simulink model "ssc_auto_ev_20b"  (R2020b)
settings: Solver=VariableStepAuto  StartTime=0.0  StopTime=200  RelTol=1e-3  AbsTol=1e-3
PreLoadFcn:
  | % Simulation parameters
  | dt = 0.01;
  | 
  | % Battery cell parameters
  | ssc_lithium_cell_1RC_ini
  | Nseries = 100;
  | Nparallel = 10;
  | 
  | % Motor parameters
  | max_torque = 220;
  | max_power = 80e3;
  | 
  | % Vehicle parameters
  | vehicle_mass = 4000;
  | wheel_radius = 0.35;
  | area = 5;
  | drag_coefficient = 0.25;
  | air_density = 1.225;
  | gravity = 9.81;
  | rolling_res_ratio = 0.015;
  | 
  | % Differential drive parameters
  | gear_ratio = 12;
  | 
  | % Simplified braking system parameters
  | force_max_pedal = 500;
  | braking_torque_to_pedal_force_ratio = -16;
  | 
  | % Vehicle controller parameters
  | hill_hold_max_speed = 0.5;
  | 
  | % Water properties for cooling circuit
  | load WaterProperties
  | 
  | % Input signals for Signal Editor block
  | load ssc_auto_ev_Inputs
values from neighbouring files (symbols this model uses):
  C1_LUT = [1913.6 4625.7 23306 10736 18036 12251 9022.9 12447 18872 40764 18721 33630 ... (21 elements, 7x3)]    [ssc_auto_ev_param.mat]
  Capacity_LUT = [28.0081 27.625 27.6392]    [ssc_auto_ev_param.mat]
  cell_Cp_heat = 810.5328    [ssc_auto_ev_param.mat]
  cell_mass = 1    [ssc_auto_ev_param.mat]
  Em_LUT = [3.4966 3.5519 3.6183 3.7066 3.9131 4.0748 4.1923 3.5057 3.566 3.6337 3.7127 3.9259 ... (21 elements, 7x3)]    [ssc_auto_ev_param.mat]
  Qe_init = 15.6845    [ssc_auto_ev_param.mat]
  R0_LUT = [0.0117 0.011 0.0114 0.0107 0.0107 0.0113 0.0116 0.0085 0.0085 0.0087 0.0082 0.0083 ... (21 elements, 7x3)]    [ssc_auto_ev_param.mat]
  R1_LUT = [0.0109 0.0069 0.0047 0.0034 0.0033 0.0033 0.0028 0.0029 0.0024 0.0026 0.0016 0.0023 ... (21 elements, 7x3)]    [ssc_auto_ev_param.mat]
  SOC_LUT = [0 0.1 0.25 0.5 0.75 0.9 1]    [ssc_auto_ev_param.mat]
  T_init = 293.15    [ssc_auto_ev_param.mat]
  Temperature_LUT = [278.15 293.15 313.15]    [ssc_auto_ev_param.mat]
undefined symbols (not defined in the file or in its folder): DiscIntNeverNeededParam, K, Lambda, tau, x0
libraries: fl_lib x656, nesl_utility x86, simulink x21, LiBatteryElements_lib x16, SignalEditorBlockLib x4, simulink_extras x4
(part 1 of 13)
CloseFcn:
  | try,close(h1_ssc_auto_ev),end
  | clear h1_ssc_auto_ev
  | 
  | clear simlog_ssc_auto_ev
  | clear logsout_ssc_auto_ev
  | clear Nseries Nparallel
  | clear C1_LUT Capacity_LUT Cp Cv
  | clear Em_LUT Qe_init R0_LUT R1_LUT
  | clear SOC_LUT T T_init Temperature_LUT
  | clear air_density alpha area beta
  | clear braking_torque_to_pedal_force_ratio
  | clear cell_Cp_heat cell_area cell_height
  | clear cell_mass cell_rho_Cp cell_thickness
  | clear cell_volume cell_width drag_coefficient
  | clear dt force_max_pedal gear_ratio gravity
  | clear h h_conv hill_hold_max_speed k
  | clear max_power max_torque nu p rho
  | clear rolling_res_ratio simlog_TMotor tout u
  | clear vehicle_mass wheel_radius Test_1
Description:
  | Configuring an EV Simulation for Multirate HIL
settings Model: Creator=The MathWorks, Inc.  LastModifiedBy=amyyang
settings SolverCC: AutoScaleAbsTol=off
settings DataIOCC: ReturnWorkspaceOutputs=off  SignalLoggingName=logsout_ssc_auto_ev
settings DebuggingCC: SymbolicDimsDataTypeCodeGenerationDiagnostic=none
settings SFSimCC: CustomCodeUndefinedFunction=UseInterfaceOnly
settings SimscapeCC: SimscapeLogType=all  SimscapeLogName=simlog_ssc_auto_ev  SimscapeLogDataHistory=40000

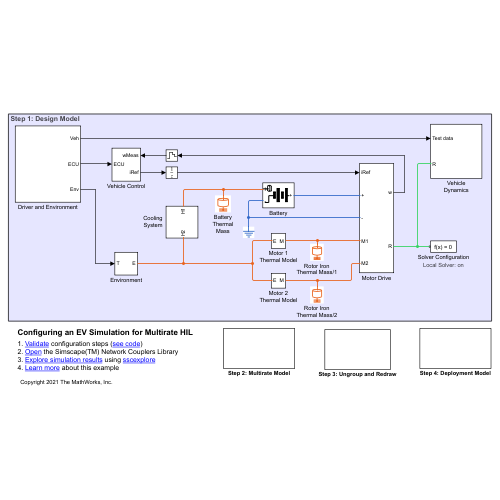
[thumbnail: Simulink's stored preview of the top-level diagram]
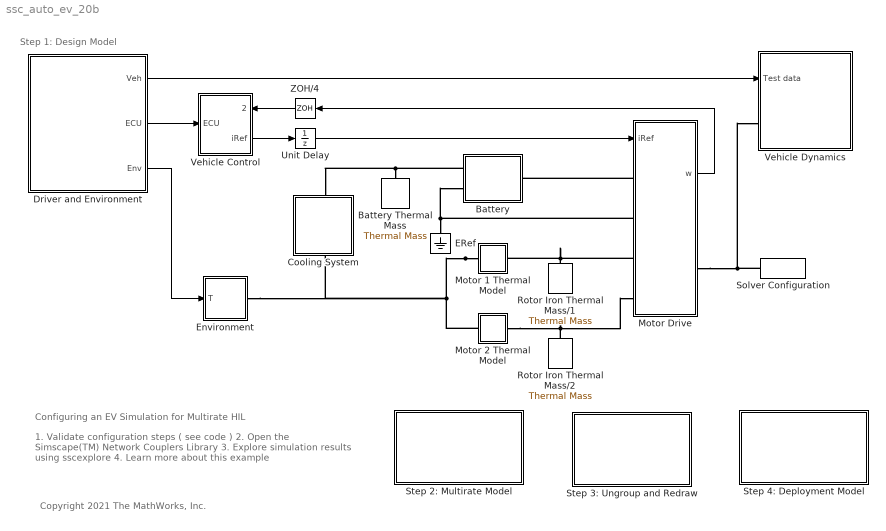
== system ssc_auto_ev_20b ==
  note: Step 1: Design Model
  note: Configuring an EV Simulation for Multirate HIL
  note: 1. Validate configuration steps ( see code )
      | 2. Open the Simscape(TM) Network Couplers Library
      | 3. Explore simulation results using sscexplore
      | 4. Learn more about this example
  note: Copyright 2021 The MathWorks, Inc.
  Battery : Subsystem  mask(Lithium cell (one RC-branch equivalent circuit)){Nseries=Nseries, Nparallel=Nparallel, Qe_init=Qe_init, Capacity_LUT=Capacity_LUT, Em_LUT=Em_LUT, R0_LUT=R0_LUT, R1_LUT=R1_LUT, C1_LUT=C1_LUT, SOC_LUT=SOC_LUT, Temperature_LUT=Temperature_LUT}
      mask prompts: Nseries "Number of series-connected parallel sets"; Nparallel "Number of parallel-connected cells per parallel set"; Qe_init "Initial cell charge deficit (A*hr)"; Capacity_LUT "Capacity (A*hr, 1xN table)"; Em_LUT "Em open-circuit voltage, Em (volts, MxN table)"; R0_LUT "R0 terminal resistance (ohms, MxN table)"; R1_LUT "R1 cell resistance (ohms, MxN table)"; C1_LUT "C1 capacitance (farads, MxN table)"; SOC_LUT "SOC table breakpoints (Mx1 array)"; Temperature_LUT "Temperature table breakpoints (K, 1xN array)"
      mask DialogControl ParameterTabVar0 Prompt: Main
      mask DialogControl ParameterTabVar01 Prompt: Electrical (per cell)
      mask DialogControl ParameterTabVar0123 Prompt: Table Breakpoints
      mask Display:
      | % Battery icon
      | plot([1.8 1.3],[0 0])
      | plot([-0.6 -1.6 -1.6 -2.2],[0 0 -0.9 -0.9])
      | patch([1 1 -1 -1]*0.15+0.7,[-1 1 1 -1]*0.4,[0;0;0]);
      | patch([1 1 -1 -1]*0.15-0.6,[-1 1 1 -1]*0.4,[0;0;0]);
      | patch([1 1 -1 -1]*0.15+1.3,[-1 1 1 -1]*0.8,[0;0;0]);
      | patch([1 1 -1 -1]*0.15-0.0,[-1 1 1 -1]*0.8,[0;0;0]);
      | % Thermal port
      | plot([-1.6,-1.3],[1.2,1.2])
      | plot([-1.6,-1.3],[0.5,0.5])
      | plot([-1.6,-2.5],[0.8,0.8])
      | plot(0.2*sin(0:2*pi/50:2*pi)-1.6,0.35*cos(0:2*pi/50:2*pi)+0.85)
      | plot(0.2*sin(0:2*pi/50:pi)-1.3,0.35*cos(0:2*pi/50:pi)+0.85)
      | 
      | % Plot points to set plot range
      | color('white');plot(2.5,1.5);plot(-2.5,-1.5)
  Battery Thermal Mass : fl_lib/Thermal/Thermal Elements/Thermal Mass  mass=cell_mass*Nseries*Nparallel kg  sp_heat=cell_Cp_heat J/(K*kg)  T_specify=on  T_priority=High  T=T_init K  T_nominal_specify=off  T_nominal_unit=K  T_nominal_value=1  Q_specify=off  Q_priority=None  Q=0 W  Q_nominal_specify=off  Q_nominal_unit=W  Q_nominal_value=1
      settings: SourceProductBaseCode=PW,SS,VE
  Cooling System : Subsystem  Tag=PublishSubsystem
      settings: PortSchema="{\"entries\":[{\"content\":{\"sides\":[{\"content\":{\"connectorIds\":[]},\"type\":\"ConnectorPlacement.EquallySpacedRectSide\",\"uuid\":\"d96bbf63-bcbb-4f3a-92bd-eaf78ab4538b\"},{\"content\":{\"connectorIds\":[],\"side\":\"RIGHT\"},\"type\":\"ConnectorPlacement.EquallySpacedRectSide\",\"uuid\":\"b082d3d3-6635-4bf9-9df2-69e4bab78a2b\"},{\"content\":{\"connectorIds\":[\"LConn1\"],\"side\":\"TOP\"},\"type\":\"ConnectorPlacement.EquallySpacedRectSide\",\"uuid\":\"f7177de9-9ba4-478b-b096-87cbc5cd4871\"},{\"content\":{\"connectorIds\":[\"RConn1\"],\"side\":\"BOTTOM\"},\"type\":\"ConnectorPlacement.EquallySpacedRectSide\",\"uuid\":\"4233a269-bfd6-4033-b1ed-0dae7bb50bca\"}]},\"type\":\"ConnectorPlacement.EquallySpacedConnector\",\"uuid\":\"6f10551f-62c9-4564-9ac9-7ef3b87c77d6\"}],\"packageUris\":[\"http://schema.mathworks.com/mf0/Connector/R2020b\"],\"version\":\"1.0\"}"
  Driver and Environment : Subsystem
  ERef : fl_lib/Electrical/Electrical Elements/Electrical Reference
      settings: SourceProductBaseCode=PW,SS,VE
  Environment : Subsystem
  Motor 1 Thermal Model : Subsystem
  Motor 2 Thermal Model : Subsystem
  Motor Drive : Subsystem  Tag=PublishSubsystem  VariantControl=Variant1
  Rotor Iron Thermal Mass/1 : fl_lib/Thermal/Thermal Elements/Thermal Mass  mass=10 kg  sp_heat=447 J/(K*kg)  T_specify=on  T_priority=High  T=T_init K  T_nominal_specify=off  T_nominal_unit=K  T_nominal_value=1  Q_specify=off  Q_priority=None  Q=0 W  Q_nominal_specify=off  Q_nominal_unit=W  Q_nominal_value=1
      settings: SourceProductBaseCode=PW,SS,VE
  Rotor Iron Thermal Mass/2 : fl_lib/Thermal/Thermal Elements/Thermal Mass  mass=10 kg  sp_heat=447 J/(K*kg)  T_specify=on  T_priority=High  T=T_init K  T_nominal_specify=off  T_nominal_unit=K  T_nominal_value=1  Q_specify=off  Q_priority=None  Q=0 W  Q_nominal_specify=off  Q_nominal_unit=W  Q_nominal_value=1
      settings: SourceProductBaseCode=PW,SS,VE
  Solver Configuration : nesl_utility/Solver Configuration  PhysicalDomain=network_engine_domain  SubClassName=solver  LeftPortType=input  RightPortType=generic  Tones=[]  Harmonics=[]  SimulateNoise=off  Profile=off  UseLocalSampling=off  EnableSwitchedLinearOptims=on  FrequencyDomain=off  UseCCode=off  RelTol=0.001  AbsTol=1e-06  MinStep=1e-09  ToWorkspace=off  RevertToSquareIcSolve=off  NumHomotopyIterations=100  PhasorMode=off  PhasorModeNumHarmonics=1  DoDC=off  ResidualTolerance=1e-9  UseLocalSolver=on  LocalSolverChoice=NE_BACKWARD_EULER_ADVANCER  LocalSolverSampleTime=dt  DoFixedCost=on  MaxNonlinIter=3  MaxModeIter=2  ComputeImpulses=off  ImpulseIterations=2  LinearAlgebra=auto  EquationFormulation=NE_TIME_EF  DelaysMemoryBudget=1024  AutomaticFiltering=on  FilteringTimeConstant=0.001  PartitionStorageMethod=AS_NEEDED  PartitionMemoryBudget=1024  PartitionMethod=FAST
      settings: AttributesFormatString=Local Solver: %<UseLocalSolver>  SourceProductBaseCode=SS,PW,VE
  Step 2: Multirate Model : Subsystem
  Step 3: Ungroup and Redraw : Subsystem
  Step 4: Deployment Model : Subsystem
  Unit Delay : UnitDelay  SampleTime=dt  HasFrameUpgradeWarning=on
  Vehicle Dynamics : Subsystem
  Vehicle Control : Subsystem  Tag=PublishSubsystem
      settings: PortSchema="{\"entries\":[{\"content\":{\"sides\":[{\"content\":{\"connectorIds\":[\"In1\"]},\"type\":\"ConnectorPlacement.EquallySpacedRectSide\",\"uuid\":\"b68a5c30-2a17-4a0c-a85e-064518f12190\"},{\"content\":{\"connectorIds\":[\"In2\",\"Out1\"],\"side\":\"RIGHT\"},\"type\":\"ConnectorPlacement.EquallySpacedRectSide\",\"uuid\":\"e14e894a-37e1-47c1-8ef8-e46ccf22e5bb\"},{\"content\":{\"connectorIds\":[],\"side\":\"TOP\"},\"type\":\"ConnectorPlacement.EquallySpacedRectSide\",\"uuid\":\"6e722464-54b7-4a5f-a776-dae3a11285e7\"}]},\"type\":\"ConnectorPlacement.EquallySpacedConnector\",\"uuid\":\"82601a10-23cc-4178-a2d7-02b0e1b6e975\"}],\"packageUris\":[\"http://schema.mathworks.com/mf0/Connector/R2020b\"],\"version\":\"1.0\"}"
  ZOH/4 : ZeroOrderHold  SampleTime=dt
  wires:
  Motor Drive/1(w) -> ZOH/4/1
  Unit Delay/1 -> Motor Drive/1(iRef)
  Vehicle Control/1(iRef) -> Unit Delay/1
  ZOH/4/1 -> Vehicle Control/2(wMeas)
  Driver and Environment/2(ECU) -> Vehicle Control/1(ECU)
  Driver and Environment/3(Env) -> Environment/1(T)
  Driver and Environment/1(Veh) -> Vehicle Dynamics/1(Test data)
  connections:
  Motor 1 Thermal Model/LConn1 -- Motor 2 Thermal Model/LConn1 -- Environment/RConn1 -- Cooling System/RConn1
  Motor Drive/LConn2 -- Battery/LConn2 -- ERef/LConn1
  Motor Drive/LConn1 -- Battery/RConn1
  Motor Drive/RConn1 -- Vehicle Dynamics/LConn1 -- Solver Configuration/RConn1
  Motor Drive/LConn3 -- Motor 1 Thermal Model/RConn1 -- Rotor Iron Thermal Mass/1/LConn1
  Battery/LConn1 -- Cooling System/LConn1 -- Battery Thermal Mass/LConn1
  Motor 2 Thermal Model/RConn1 -- Rotor Iron Thermal Mass/2/LConn1 -- Motor Drive/LConn4

== system ssc_auto_ev_20b/Battery ==
  note: Scale up voltage drop to total
      | of Ns series-connected cells
  Controlled Voltage Source : fl_lib/Electrical/Electrical Sources/Controlled Voltage Source
      settings: SourceProductBaseCode=PW,SS,VE
  Electric and Thermal Model : Subsystem  Tag=PublishSubsystem
  Nseries-1 : fl_lib/Physical Signals/Functions/PS Gain  gain=Nseries-1
      settings: SourceProductBaseCode=PW,SS,VE
  PS Terminator : fl_lib/Physical Signals/Sinks/PS Terminator
      settings: SourceProductBaseCode=PW,SS,VE
  Temperature Sensor : fl_lib/Thermal/Thermal Sensors/Temperature Sensor
      settings: SourceProductBaseCode=PW,SS,VE
  Thermal Reference : fl_lib/Thermal/Thermal Elements/Thermal Reference
      settings: SourceProductBaseCode=PW,SS,VE
  Voltage Sensor : fl_lib/Electrical/Electrical Sensors/Voltage Sensor
      settings: SourceProductBaseCode=PW,SS,VE
  + : PMIOPort  Tag=PMCPort  Side=Right
  H : PMIOPort  Tag=PMCPort  Port=2  Side=Left
  - : PMIOPort  Tag=PMCPort  Port=3  Side=Left
  connections:
  H/RConn1 -- Temperature Sensor/LConn1 -- Electric and Thermal Model/LConn1
  Controlled Voltage Source/LConn1 -- Voltage Sensor/RConn2 -- Electric and Thermal Model/RConn2
  Nseries-1/LConn1 -- Voltage Sensor/RConn1
  Voltage Sensor/LConn1 -- Electric and Thermal Model/RConn1 -- +/RConn1
  Nseries-1/RConn1 -- Controlled Voltage Source/RConn1
  Controlled Voltage Source/RConn2 -- -/RConn1
  Temperature Sensor/RConn1 -- Thermal Reference/LConn1
  PS Terminator/LConn1 -- Temperature Sensor/RConn2

== system ssc_auto_ev_20b/Cooling System ==
  note: Radiator
  note: Battery Heat Exchanger
  " Heat Exchanger Characteristic" : Subsystem
  Convection Battery-Env : fl_lib/Thermal/Thermal Elements/Convective Heat Transfer  area=cell_area m^2  heat_tr_coeff=h_conv W/(m^2 * K)  T_specify=off  T_priority=High  T=0 K  T_nominal_specify=off  T_nominal_unit=K  T_nominal_value=1  Q_specify=off  Q_priority=High  Q=0 J/s  Q_nominal_specify=off  Q_nominal_unit=J/s  Q_nominal_value=1
      settings: SourceProductBaseCode=PW,SS,VE
  Expansion Tank : Subsystem
  Heat Exchanger Characteristic : Subsystem
  Hose Radiator : fl_lib/Thermal Liquid/Elements/Pipe (TL)  length=2000 mm  area=pi*25^2 mm^2  Dh=50 mm  length_add=500 mm  roughness=1.5e-5 m  Re_lam=2e+3  Re_tur=4e+3  shape_factor=64  Nu_lam=3.66  dynamic_compressibility=1  inertia=0  p0=1 atm  T0=20 degC  mdot0=0.1 kg/s
      settings: SourceProductBaseCode=PW,SS,VE
  Hose Inlet : fl_lib/Thermal Liquid/Elements/Pipe (TL)  length=500 mm  area=pi*25^2 mm^2  Dh=50 mm  length_add=500 mm  roughness=1.5e-5 m  Re_lam=2e+3  Re_tur=4e+3  shape_factor=64  Nu_lam=3.66  dynamic_compressibility=1  inertia=0  p0=1 atm  T0=20 degC  mdot0=0.1 kg/s
      settings: SourceProductBaseCode=PW,SS,VE
  Hose Outlet : fl_lib/Thermal Liquid/Elements/Pipe (TL)  length=500 mm  area=pi*25^2 mm^2  Dh=50 mm  length_add=500 mm  roughness=1.5e-5 m  Re_lam=2e+3  Re_tur=4e+3  shape_factor=64  Nu_lam=3.66  dynamic_compressibility=1  inertia=0  p0=1 atm  T0=20 degC  mdot0=0.1 kg/s
      settings: SourceProductBaseCode=PW,SS,VE
  Insulator Inlet Hose : fl_lib/Thermal/Thermal Elements/Perfect Insulator  T_specify=off  T_priority=High  T=0 K  T_nominal_specify=off  T_nominal_unit=K  T_nominal_value=1
      settings: SourceProductBaseCode=PW,SS,VE
  Insulator Outlet Hose : fl_lib/Thermal/Thermal Elements/Perfect Insulator  T_specify=off  T_priority=High  T=0 K  T_nominal_specify=off  T_nominal_unit=K  T_nominal_value=1
      settings: SourceProductBaseCode=PW,SS,VE
  PS Terminator : fl_lib/Physical Signals/Sinks/PS Terminator
      settings: SourceProductBaseCode=PW,SS,VE
  Pipe : fl_lib/Thermal Liquid/Elements/Pipe (TL)  length=400 mm  area=pi*25^2 mm^2  Dh=50 mm  length_add=500 mm  roughness=1.5e-5 m  Re_lam=2e+3  Re_tur=4e+3  shape_factor=64  Nu_lam=3.66  dynamic_compressibility=1  inertia=0  p0=1 atm  T0=20 degC  mdot0=0.1 kg/s
      settings: SourceProductBaseCode=PW,SS,VE
  Pump : fl_lib/Thermal Liquid/Sources/Mass Flow Rate Source (TL)  commanded_mass_flow=0.2 kg/s  area=pi*25^2 mm^2
      settings: SourceProductBaseCode=PW,SS,VE  InternalSimscapePortConfiguration="{\"Bottom\":[],\"Left\":[{\"id\":\"A\",\"label\":\"A\",\"type\":\"foundation.thermal_liquid.thermal_liquid\"}],\"Right\":[{\"id\":\"B\",\"label\":\"B\",\"type\":\"foundation.thermal_liquid.thermal_liquid\"}],\"Top\":[]}"
  Sensing Inlet Temperature : Subsystem
      mask Display: disp('T');
  Sensing Temperature : Subsystem
      mask Display: disp('T')
  Thermal Liquid Settings (TL) : fl_lib/Thermal Liquid/Utilities/Thermal Liquid Settings (TL)  table_dimensions=0  T_TLU=T K  p_TLU=p Pa  p_atm=1 atm  pT_region_flag=0  T_min=273.16 K  T_max=373.16 K  p_min=0.1 bar  p_max=500 bar  T_min_1D=273.16 K  T_max_1D=373.16 K  p_min_1D=0.01 MPa  p_max_1D=50 MPa  pT_validity_TLU=ones(11, 12)  rho_parameterization_2D=1  rho_parameterization_1D=1  rho_TLU=rho kg/m^3  beta_TLU=beta Pa  alpha_TLU=alpha 1/K  rho_TLU_2=[999.7973, 999.8431, 1002.3216, 1004.8218, 1007.293, 1009.7358, 1012.1506, 1014.5379, 1016.8979, 1019.2311, 1021.538, 1023.8188; 999.6579, 999.7009, 1002.0303, 1004.382, 1006.7084, 1009.0101, 1011.2874, 1013.5407, 1015.7703, 1017.9766, 1020.1599, 1022.3206; 998.1632, 998.2045, 1000.4375, 1002.6924, 1004.9239, 1007.1324, 1009.3183, 1011.4819, 1013.6236, 1015.7438, 1017.8428, 1019.921; 995.6057, 995.6458, 997.81864, 1000.0128, 1002.1841, 1004.3332, 1006.4603, 1008.566, 1010.6505, 1012.7144, 1014.758, 1016.7815; 992.1724, 992.2119, 994.35133, 996.5113, 998.6484, 1000.7633, 1002.8563, 1004.928, 1006.9788, 1009.009, 1011.0192, 1013.0097; 988.02, 988.0299, 990.15684, 992.3035, 994.4268, 996.5273, 998.6056, 1000.6622, 1002.6976, 1004.7123, 1006.7067, 1008.6813; 983.18, 983.1901, 985.3217, 987.4721, 989.5983, 991.7008, 993.7803, 995.8374, 997.8726, 999.8864, 1001.8795, 1003.8522; 977.75, 977.7583, 979.9094, 982.0783, 984.2216, 986.34, 988.4343, 990.505, 992.5529, 994.5786, 996.5825, 998.5654; 971.77, 971.7836, 973.96734, 976.1678, 978.3409, 980.4876, 982.6087, 984.7049, 986.7768, 988.8254, 990.8511, 992.8545; 965.26, 965.3023, 967.53107, 969.7753, 971.9901, 974.1764, 976.3354, 978.4676, 980.5741, 982.6556, 984.7129, 986.7465; 958.62, 958.6315, 960.627, 962.9267, 965.1944, 967.4314, 969.6387, 971.8173, 973.9681, 976.0921, 978.19, 980.2628] kg/m^3  rho_ref_3=998.21 kg/m^3  T_ref_3=293.16 K  p_ref_3=0.101325 MPa  beta_const_3=2.1791 GPa  alpha_const_3=2.0691e-4 1/K  rho_TLU_4=[999.84; 999.7; 998.2; 995.65; 992.21; 988.03; 983.19; 977.76; 971.78; 965.3; 958.8] kg/m^3  beta_const_4=2.1791 GPa  p_ref_4=0.101325 MPa  rho_ref_5=998.21 kg/m^3  T_ref_5=293.16 K  p_ref_5=0.101325 MPa  beta_const_5=2.1791 GPa  alpha_const_5=2.0691e-4 1/K  u_parameterization_2D=1  u_parameterization_1D=1  u_TLU=u J/g  cp_TLU=Cp J/K/g  u_TLU_2=[.0002, .0018, .086, .1588, .219, .267, .3034, .3288, .3436, .3483, .3435, .3294; 42.062, 42.06, 41.935, 41.804, 41.668, 41.527, 41.382, 41.233, 41.081, 40.924, 40.763, 40.599; 83.953, 83.948, 83.651, 83.349, 83.049, 82.749, 82.451, 82.153, 81.856, 81.56, 81.265, 80.971; 125.77, 125.76, 125.31, 124.86, 124.41, 123.97, 123.53, 123.1, 122.68, 122.25, 121.84, 121.42; 167.57, 167.56, 166.96, 166.37, 165.79, 165.21, 164.65, 164.09, 163.54, 163, 162.46, 161.94; 209.36, 209.36, 208.63, 207.9, 207.19, 206.48, 205.79, 205.11, 204.45, 203.79, 203.14, 202.5; 251.19, 251.19, 250.33, 249.47, 248.62, 247.79, 246.98, 246.18, 245.39, 244.62, 243.86, 243.12; 293.06, 293.06, 292.07, 291.07, 290.1, 289.14, 288.2, 287.28, 286.38, 285.49, 284.62, 283.77; 334.99, 334.99, 333.86, 332.73, 331.63, 330.54, 329.48, 328.44, 327.41, 326.41, 325.43, 324.46; 377, 377, 375.73, 374.46, 373.22, 372, 370.81, 369.64, 368.5, 367.38, 366.27, 365.19; 419.01, 419.01, 417.69, 416.27, 414.89, 413.54, 412.21, 410.91, 409.64, 408.4, 407.17, 405.98] kJ/kg  cp_TLU_3=[4.2199, 4.2194, 4.1957, 4.1726, 4.1508, 4.13, 4.1103, 4.0916, 4.0738, 4.0569, 4.0408, 4.0254; 4.1955, 4.1951, 4.1769, 4.1592, 4.1422, 4.1259, 4.1103, 4.0954, 4.0812, 4.0676, 4.0545, 4.0421; 4.1843, 4.184, 4.169, 4.1543, 4.1401, 4.1264, 4.1133, 4.1007, 4.0885, 4.0768, 4.0656, 4.0548; 4.1801, 4.1798, 4.1667, 4.1538, 4.1413, 4.1293, 4.1177, 4.1064, 4.0956, 4.0851, 4.075, 4.0653; 4.1796, 4.1794, 4.1675, 4.1558, 4.1444, 4.1334, 4.1227, 4.1123, 4.1023, 4.0926, 4.0832, 4.0741; 4.1813, 4.1813, 4.1702, 4.1592, 4.1484, 4.138, 4.1279, 4.1181, 4.1086, 4.0993, 4.0903, 4.0816; 4.185, 4.185, 4.1742, 4.1636, 4.1532, 4.1432, 4.1334, 4.1239, 4.1146, 4.1056, 4.0969, 4.0884; 4.1901, 4.1901, 4.1795, 4.169, 4.1588, 4.1489, 4.1393, 4.1299, 4.1207, 4.1118, 4.1032, 4.0947; 4.1968, 4.1968, 4.1862, 4.1757, 4.1655, 4.1555, 4.1458, 4.1364, 4.1273, 4.1183, 4.1096, 4.1012; 4.2052, 4.2052, 4.1944, 4.1837, 4.1733, 4.1632, 4.1534, 4.1438, 4.1345, 4.1255, 4.1166, 4.108; 4.2136, 4.2136, 4.2045, 4.1935, 4.1828, 4.1724, 4.1623, 4.1524, 4.1429, 4.1335, 4.1245, 4.1157] kJ/kg/K  u_TLU_4=[.0018; 42.06; 83.948; 125.76; 167.56; 209.36; 251.19; 293.06; 334.99; 377; 418.01] kJ/kg  cp_TLU_5=[4.2199; 4.1955; 4.1843; 4.1801; 4.1796; 4.1813; 4.185; 4.1901; 4.1968; 4.2052; 4.2136] kJ/kg/K  nu_TLU=nu cm^2/s  nu_TLU_2=[1.7917; 1.3061; 1.0032; .8006; .6577; .553; .4739; .4127; .3643; .3254; .2866] mm^2/s  k_TLU=k mW/m/K  k_TLU_2=[561.04; 580.02; 598.44; 615.48; 630.6; 643.61; 654.39; 663.13; 670.02; 675.27; 680.52] mW/m/K
      settings: SourceProductBaseCode=PW,SS,VE
  H1 : PMIOPort  Side=Left
  H2 : PMIOPort  Port=2  Side=Right
  connections:
  PS Terminator/LConn1 -- " Heat Exchanger Characteristic"/RConn3
  Sensing Temperature/RConn1 -- " Heat Exchanger Characteristic"/LConn3
  " Heat Exchanger Characteristic"/LConn1 -- Hose Radiator/LConn2
  Hose Radiator/LConn1 -- " Heat Exchanger Characteristic"/LConn2
  Hose Inlet/LConn1 -- Hose Radiator/RConn1 -- Sensing Temperature/LConn1
  Hose Outlet/LConn1 -- " Heat Exchanger Characteristic"/RConn2
  Pump/LConn1 -- Hose Outlet/RConn1 -- Thermal Liquid Settings (TL)/RConn1
  H2/RConn1 -- " Heat Exchanger Characteristic"/RConn1 -- Convection Battery-Env/LConn1
  Insulator Inlet Hose/LConn1 -- Hose Inlet/LConn2
  Insulator Outlet Hose/LConn1 -- Hose Outlet/LConn2
  Pipe/RConn1 -- Pump/RConn1 -- Sensing Inlet Temperature/LConn1
  Heat Exchanger Characteristic/LConn1 -- Pipe/LConn2
  Heat Exchanger Characteristic/RConn1 -- H1/RConn1 -- Convection Battery-Env/RConn1
  Pipe/LConn1 -- Heat Exchanger Characteristic/LConn2
  Heat Exchanger Characteristic/LConn3 -- Sensing Inlet Temperature/RConn1
  Expansion Tank/LConn1 -- Heat Exchanger Characteristic/RConn2 -- Hose Inlet/RConn1

== system ssc_auto_ev_20b/Driver and Environment ==
  Bus : Subsystem
  Bus Creator : BusCreator  Inputs=5
  Inclinometer : Subsystem
  Inputs : SignalEditorBlockLib/Signal Editor  FileName=ssc_auto_ev_Inputs.mat  ActiveScenario=Test_1  ActiveSignal=Env (deg C)  IsBus=off  OutputBusObjectStr=Bus: BusObject  SampleTime=0.01  OutputAfterFinalValue=Extrapolation  Unit=inherit  PreserveSignalName=on
  ZOH/{2..3,5..7} (5 alike) : ZeroOrderHold  SampleTime=dt
  Veh : Outport
  ECU : Outport  Port=2
  Env : Outport  Port=3
  wires:
  ? -> Bus/2(Wi)
  Inclinometer/1(y) -> ZOH/6/1
  ? -> ZOH/2/1
  ? -> ZOH/3/1
  Inputs/1 -> Inclinometer/1(a), Bus/1(In)
  ? -> ZOH/7/1
  ? -> Env/1
  Bus/1(b) -> Veh/1
  Bus Creator/1 -> ECU/1
  ZOH/5/1 -> Bus Creator/2  "Brake pedal"
  ZOH/2/1 -> Bus Creator/3  "Throttle"
  ZOH/3/1 -> Bus Creator/4  "Cruise enable"
  ZOH/7/1 -> Bus Creator/5  "Cruise disable"
  ZOH/6/1 -> Bus Creator/1  "Incline"
  ? -> Bus/3(Br), ZOH/5/1

== system ssc_auto_ev_20b/Environment ==
  T : Inport
  Ambient Temperature : fl_lib/Thermal/Thermal Sources/Controlled Temperature Source
      settings: SourceProductBaseCode=PW,SS,VE
  Simulink-PS Converter1 : nesl_utility/Simulink-PS Converter  PhysicalDomain=network_engine_domain  SubClassName=ps_input  LeftPortType=input  RightPortType=output  PseudoPeriodic=off  Frequencies=[]  NoiseDistribution=none  NoiseParameters=[]  Unit=degC  AffineConversion=on  FilteringAndDerivatives=zero  SimscapeFilterOrder=1  InputFilterTimeConstant=.001  UdotUserProvided=1
      settings: SourceProductBaseCode=SS,PW,VE
  ThRef1 : fl_lib/Thermal/Thermal Elements/Thermal Reference
      settings: SourceProductBaseCode=PW,SS,VE
  E : PMIOPort  Side=Right
  wires:
  T/1 -> Simulink-PS Converter1/1
  connections:
  Ambient Temperature/RConn2 -- ThRef1/LConn1
  Ambient Temperature/RConn1 -- Simulink-PS Converter1/RConn1
  Ambient Temperature/LConn1 -- E/RConn1

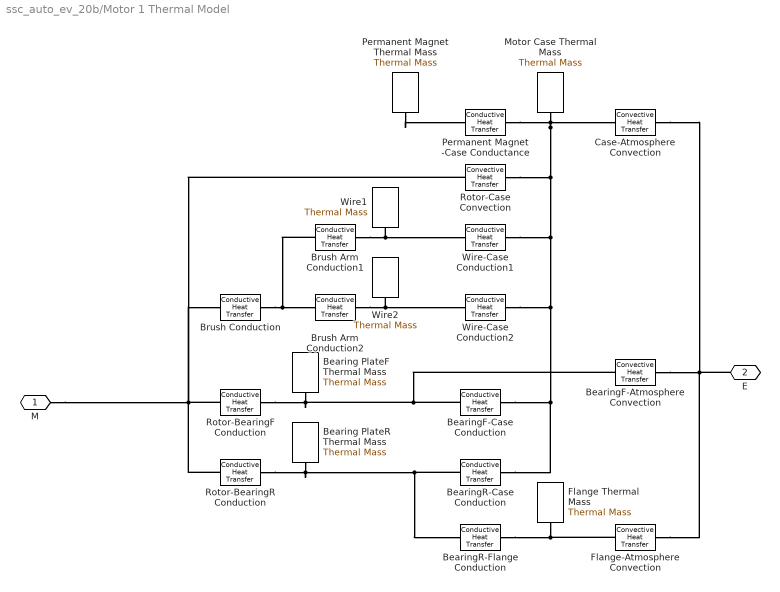
== system ssc_auto_ev_20b/Motor 1 Thermal Model ==
  Bearing PlateF Thermal Mass : fl_lib/Thermal/Thermal Elements/Thermal Mass  mass=0.6 kg  sp_heat=447 J/kg/K  T_specify=off  T_priority=High  T=300 K  T_nominal_specify=off  T_nominal_unit=K  T_nominal_value=1  Q_specify=off  Q_priority=None  Q=0 W  Q_nominal_specify=off  Q_nominal_unit=W  Q_nominal_value=1
      settings: SourceProductBaseCode=PW,SS,VE
  Bearing PlateR Thermal Mass : fl_lib/Thermal/Thermal Elements/Thermal Mass  mass=0.6 kg  sp_heat=447 J/kg/K  T_specify=off  T_priority=High  T=300 K  T_nominal_specify=off  T_nominal_unit=K  T_nominal_value=1  Q_specify=off  Q_priority=None  Q=0 W  Q_nominal_specify=off  Q_nominal_unit=W  Q_nominal_value=1
      settings: SourceProductBaseCode=PW,SS,VE
  BearingF-Atmosphere Convection : fl_lib/Thermal/Thermal Elements/Convective Heat Transfer  area=274.6 cm^2  heat_tr_coeff=123.5 W/(m^2 * K)  T_specify=off  T_priority=None  T=0 K  T_nominal_specify=off  T_nominal_unit=K  T_nominal_value=1  Q_specify=off  Q_priority=None  Q=0 W  Q_nominal_specify=off  Q_nominal_unit=W  Q_nominal_value=1
      settings: SourceProductBaseCode=PW,SS,VE
  BearingF-Case Conduction : fl_lib/Thermal/Thermal Elements/Conductive Heat Transfer  area=145 cm^2  thickness=18 cm  th_cond=80.2 W/(m*K)  T_specify=off  T_priority=None  T=0 K  T_nominal_specify=off  T_nominal_unit=K  T_nominal_value=1  Q_specify=off  Q_priority=None  Q=0 W  Q_nominal_specify=off  Q_nominal_unit=W  Q_nominal_value=1
      settings: SourceProductBaseCode=PW,SS,VE
  BearingR-Case Conduction : fl_lib/Thermal/Thermal Elements/Conductive Heat Transfer  area=145 cm^2  thickness=25 cm  th_cond=80.2 W/(m*K)  T_specify=off  T_priority=None  T=0 K  T_nominal_specify=off  T_nominal_unit=K  T_nominal_value=1  Q_specify=off  Q_priority=None  Q=0 W  Q_nominal_specify=off  Q_nominal_unit=W  Q_nominal_value=1
      settings: SourceProductBaseCode=PW,SS,VE
  BearingR-Flange Conduction : fl_lib/Thermal/Thermal Elements/Conductive Heat Transfer  area=34.5 cm^2  thickness=14 cm  th_cond=80.2 W/(m*K)  T_specify=off  T_priority=None  T=0 K  T_nominal_specify=off  T_nominal_unit=K  T_nominal_value=1  Q_specify=off  Q_priority=None  Q=0 W  Q_nominal_specify=off  Q_nominal_unit=W  Q_nominal_value=1
      settings: SourceProductBaseCode=PW,SS,VE
  Brush Conduction : fl_lib/Thermal/Thermal Elements/Conductive Heat Transfer  area=3*5 cm^2  thickness=4 cm  th_cond=1.7 W/(m*K)  T_specify=off  T_priority=None  T=0 K  T_nominal_specify=off  T_nominal_unit=K  T_nominal_value=1  Q_specify=off  Q_priority=None  Q=0 W  Q_nominal_specify=off  Q_nominal_unit=W  Q_nominal_value=1
      settings: SourceProductBaseCode=PW,SS,VE
  Brush Arm Conduction1 : fl_lib/Thermal/Thermal Elements/Conductive Heat Transfer  area=3*5 cm^2  thickness=4 cm  th_cond=1.7 W/(m*K)  T_specify=off  T_priority=None  T=0 K  T_nominal_specify=off  T_nominal_unit=K  T_nominal_value=1  Q_specify=off  Q_priority=None  Q=0 W  Q_nominal_specify=off  Q_nominal_unit=W  Q_nominal_value=1
      settings: SourceProductBaseCode=PW,SS,VE
  Brush Arm Conduction2 : fl_lib/Thermal/Thermal Elements/Conductive Heat Transfer  area=3*5 cm^2  thickness=4 cm  th_cond=1.7 W/(m*K)  T_specify=off  T_priority=None  T=0 K  T_nominal_specify=off  T_nominal_unit=K  T_nominal_value=1  Q_specify=off  Q_priority=None  Q=0 W  Q_nominal_specify=off  Q_nominal_unit=W  Q_nominal_value=1
      settings: SourceProductBaseCode=PW,SS,VE
  Case-Atmosphere Convection : fl_lib/Thermal/Thermal Elements/Convective Heat Transfer  area=4240 cm^2  heat_tr_coeff=26.8 W/(m^2 * K)  T_specify=off  T_priority=None  T=0 K  T_nominal_specify=off  T_nominal_unit=K  T_nominal_value=1  Q_specify=off  Q_priority=None  Q=0 W  Q_nominal_specify=off  Q_nominal_unit=W  Q_nominal_value=1
      settings: SourceProductBaseCode=PW,SS,VE
  Flange Thermal Mass : fl_lib/Thermal/Thermal Elements/Thermal Mass  mass=1.6 kg  sp_heat=447 J/kg/K  T_specify=off  T_priority=High  T=300 K  T_nominal_specify=off  T_nominal_unit=K  T_nominal_value=1  Q_specify=off  Q_priority=None  Q=0 W  Q_nominal_specify=off  Q_nominal_unit=W  Q_nominal_value=1
      settings: SourceProductBaseCode=PW,SS,VE
  Flange-Atmosphere Convection : fl_lib/Thermal/Thermal Elements/Convective Heat Transfer  area=324 cm^2  heat_tr_coeff=123.4 W/(m^2 * K)  T_specify=off  T_priority=None  T=0 K  T_nominal_specify=off  T_nominal_unit=K  T_nominal_value=1  Q_specify=off  Q_priority=None  Q=0 W  Q_nominal_specify=off  Q_nominal_unit=W  Q_nominal_value=1
      settings: SourceProductBaseCode=PW,SS,VE
  Motor Case Thermal Mass : fl_lib/Thermal/Thermal Elements/Thermal Mass  mass=3.8 kg  sp_heat=903 J/kg/K  T_specify=off  T_priority=High  T=300 K  T_nominal_specify=off  T_nominal_unit=K  T_nominal_value=1  Q_specify=off  Q_priority=None  Q=0 W  Q_nominal_specify=off  Q_nominal_unit=W  Q_nominal_value=1
      settings: SourceProductBaseCode=PW,SS,VE
  Permanent Magnet Thermal Mass : fl_lib/Thermal/Thermal Elements/Thermal Mass  mass=3.6 kg  sp_heat=447 J/kg/K  T_specify=off  T_priority=High  T=300 K  T_nominal_specify=off  T_nominal_unit=K  T_nominal_value=1  Q_specify=off  Q_priority=None  Q=0 W  Q_nominal_specify=off  Q_nominal_unit=W  Q_nominal_value=1
      settings: SourceProductBaseCode=PW,SS,VE
  Permanent Magnet -Case Conductance : fl_lib/Thermal/Thermal Elements/Conductive Heat Transfer  area=4350 cm^2  thickness=26 cm  th_cond=80.2 W/(m*K)  T_specify=off  T_priority=None  T=0 K  T_nominal_specify=off  T_nominal_unit=K  T_nominal_value=1  Q_specify=off  Q_priority=None  Q=0 W  Q_nominal_specify=off  Q_nominal_unit=W  Q_nominal_value=1
      settings: SourceProductBaseCode=PW,SS,VE
  Rotor-BearingF Conduction : fl_lib/Thermal/Thermal Elements/Conductive Heat Transfer  area=26.4 cm^2  thickness=2.5 cm  th_cond=80.2 W/(m*K)  T_specify=off  T_priority=None  T=0 K  T_nominal_specify=off  T_nominal_unit=K  T_nominal_value=1  Q_specify=off  Q_priority=None  Q=0 W  Q_nominal_specify=off  Q_nominal_unit=W  Q_nominal_value=1
      settings: SourceProductBaseCode=PW,SS,VE
  Rotor-BearingR Conduction : fl_lib/Thermal/Thermal Elements/Conductive Heat Transfer  area=26.4 cm^2  thickness=2.5 cm  th_cond=80.2 W/(m*K)  T_specify=off  T_priority=None  T=0 K  T_nominal_specify=off  T_nominal_unit=K  T_nominal_value=1  Q_specify=off  Q_priority=None  Q=0 W  Q_nominal_specify=off  Q_nominal_unit=W  Q_nominal_value=1
      settings: SourceProductBaseCode=PW,SS,VE
  Rotor-Case Convection : fl_lib/Thermal/Thermal Elements/Convective Heat Transfer  area=1240 cm^2  heat_tr_coeff=210 W/(m^2 * K)  T_specify=off  T_priority=None  T=0 K  T_nominal_specify=off  T_nominal_unit=K  T_nominal_value=1  Q_specify=off  Q_priority=None  Q=0 W  Q_nominal_specify=off  Q_nominal_unit=W  Q_nominal_value=1
      settings: SourceProductBaseCode=PW,SS,VE
  Wire-Case Conduction1 : fl_lib/Thermal/Thermal Elements/Conductive Heat Transfer  area=1 cm^2  thickness=0.2 cm  th_cond=4 W/(m*K)  T_specify=off  T_priority=None  T=0 K  T_nominal_specify=off  T_nominal_unit=K  T_nominal_value=1  Q_specify=off  Q_priority=None  Q=0 W  Q_nominal_specify=off  Q_nominal_unit=W  Q_nominal_value=1
      settings: SourceProductBaseCode=PW,SS,VE
  Wire-Case Conduction2 : fl_lib/Thermal/Thermal Elements/Conductive Heat Transfer  area=1 cm^2  thickness=0.2 cm  th_cond=4 W/(m*K)  T_specify=off  T_priority=None  T=0 K  T_nominal_specify=off  T_nominal_unit=K  T_nominal_value=1  Q_specify=off  Q_priority=None  Q=0 W  Q_nominal_specify=off  Q_nominal_unit=W  Q_nominal_value=1
      settings: SourceProductBaseCode=PW,SS,VE
  Wire1 : fl_lib/Thermal/Thermal Elements/Thermal Mass  mass=0.05 kg  sp_heat=385 J/kg/K  T_specify=off  T_priority=High  T=300 K  T_nominal_specify=off  T_nominal_unit=K  T_nominal_value=1  Q_specify=off  Q_priority=None  Q=0 W  Q_nominal_specify=off  Q_nominal_unit=W  Q_nominal_value=1
      settings: SourceProductBaseCode=PW,SS,VE
  Wire2 : fl_lib/Thermal/Thermal Elements/Thermal Mass  mass=0.05 kg  sp_heat=385 J/kg/K  T_specify=off  T_priority=High  T=300 K  T_nominal_specify=off  T_nominal_unit=K  T_nominal_value=1  Q_specify=off  Q_priority=None  Q=0 W  Q_nominal_specify=off  Q_nominal_unit=W  Q_nominal_value=1
      settings: SourceProductBaseCode=PW,SS,VE
  M : PMIOPort  Side=Right
  E : PMIOPort  Port=2  Side=Left
  connections:
  Flange-Atmosphere Convection/RConn1 -- E/RConn1 -- BearingF-Atmosphere Convection/RConn1 -- Case-Atmosphere Convection/RConn1
  Motor Case Thermal Mass/LConn1 -- Case-Atmosphere Convection/LConn1 -- Permanent Magnet -Case Conductance/RConn1 -- Wire-Case Conduction1/RConn1 -- Wire-Case Conduction2/RConn1 -- BearingF-Case Conduction/RConn1 -- BearingR-Case Conduction/RConn1 -- Rotor-Case Convection/RConn1
  Rotor-BearingR Conduction/RConn1 -- Bearing PlateR Thermal Mass/LConn1 -- BearingR-Flange Conduction/LConn1 -- BearingR-Case Conduction/LConn1
  Flange-Atmosphere Convection/LConn1 -- BearingR-Flange Conduction/RConn1 -- Flange Thermal Mass/LConn1
  BearingF-Case Conduction/LConn1 -- BearingF-Atmosphere Convection/LConn1 -- Rotor-BearingF Conduction/RConn1 -- Bearing PlateF Thermal Mass/LConn1
  Rotor-Case Convection/LConn1 -- Brush Conduction/LConn1 -- M/RConn1 -- Rotor-BearingF Conduction/LConn1 -- Rotor-BearingR Conduction/LConn1
  Permanent Magnet Thermal Mass/LConn1 -- Permanent Magnet -Case Conductance/LConn1
  Brush Conduction/RConn1 -- Brush Arm Conduction1/LConn1 -- Brush Arm Conduction2/LConn1
  Brush Arm Conduction1/RConn1 -- Wire-Case Conduction1/LConn1 -- Wire1/LConn1
  Brush Arm Conduction2/RConn1 -- Wire-Case Conduction2/LConn1 -- Wire2/LConn1

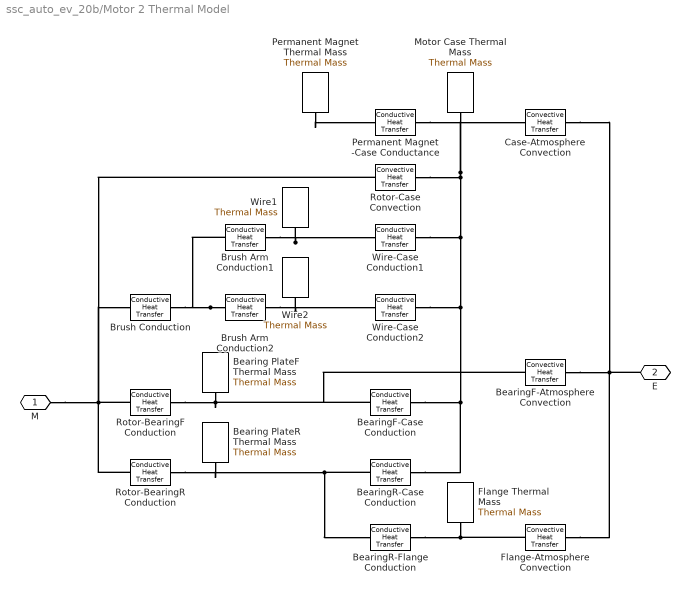
== system ssc_auto_ev_20b/Motor 2 Thermal Model ==
  Bearing PlateF Thermal Mass : fl_lib/Thermal/Thermal Elements/Thermal Mass  mass=0.6 kg  sp_heat=447 J/kg/K  T_specify=off  T_priority=High  T=300 K  T_nominal_specify=off  T_nominal_unit=K  T_nominal_value=1  Q_specify=off  Q_priority=None  Q=0 W  Q_nominal_specify=off  Q_nominal_unit=W  Q_nominal_value=1
      settings: SourceProductBaseCode=PW,SS,VE
  Bearing PlateR Thermal Mass : fl_lib/Thermal/Thermal Elements/Thermal Mass  mass=0.6 kg  sp_heat=447 J/kg/K  T_specify=off  T_priority=High  T=300 K  T_nominal_specify=off  T_nominal_unit=K  T_nominal_value=1  Q_specify=off  Q_priority=None  Q=0 W  Q_nominal_specify=off  Q_nominal_unit=W  Q_nominal_value=1
      settings: SourceProductBaseCode=PW,SS,VE
  BearingF-Atmosphere Convection : fl_lib/Thermal/Thermal Elements/Convective Heat Transfer  area=274.6 cm^2  heat_tr_coeff=123.5 W/(m^2 * K)  T_specify=off  T_priority=None  T=0 K  T_nominal_specify=off  T_nominal_unit=K  T_nominal_value=1  Q_specify=off  Q_priority=None  Q=0 W  Q_nominal_specify=off  Q_nominal_unit=W  Q_nominal_value=1
      settings: SourceProductBaseCode=PW,SS,VE
  BearingF-Case Conduction : fl_lib/Thermal/Thermal Elements/Conductive Heat Transfer  area=145 cm^2  thickness=18 cm  th_cond=80.2 W/(m*K)  T_specify=off  T_priority=None  T=0 K  T_nominal_specify=off  T_nominal_unit=K  T_nominal_value=1  Q_specify=off  Q_priority=None  Q=0 W  Q_nominal_specify=off  Q_nominal_unit=W  Q_nominal_value=1
      settings: SourceProductBaseCode=PW,SS,VE
  BearingR-Case Conduction : fl_lib/Thermal/Thermal Elements/Conductive Heat Transfer  area=145 cm^2  thickness=25 cm  th_cond=80.2 W/(m*K)  T_specify=off  T_priority=None  T=0 K  T_nominal_specify=off  T_nominal_unit=K  T_nominal_value=1  Q_specify=off  Q_priority=None  Q=0 W  Q_nominal_specify=off  Q_nominal_unit=W  Q_nominal_value=1
      settings: SourceProductBaseCode=PW,SS,VE
  BearingR-Flange Conduction : fl_lib/Thermal/Thermal Elements/Conductive Heat Transfer  area=34.5 cm^2  thickness=14 cm  th_cond=80.2 W/(m*K)  T_specify=off  T_priority=None  T=0 K  T_nominal_specify=off  T_nominal_unit=K  T_nominal_value=1  Q_specify=off  Q_priority=None  Q=0 W  Q_nominal_specify=off  Q_nominal_unit=W  Q_nominal_value=1
      settings: SourceProductBaseCode=PW,SS,VE
  Brush Conduction : fl_lib/Thermal/Thermal Elements/Conductive Heat Transfer  area=3*5 cm^2  thickness=4 cm  th_cond=1.7 W/(m*K)  T_specify=off  T_priority=None  T=0 K  T_nominal_specify=off  T_nominal_unit=K  T_nominal_value=1  Q_specify=off  Q_priority=None  Q=0 W  Q_nominal_specify=off  Q_nominal_unit=W  Q_nominal_value=1
      settings: SourceProductBaseCode=PW,SS,VE
  Brush Arm Conduction1 : fl_lib/Thermal/Thermal Elements/Conductive Heat Transfer  area=3*5 cm^2  thickness=4 cm  th_cond=1.7 W/(m*K)  T_specify=off  T_priority=None  T=0 K  T_nominal_specify=off  T_nominal_unit=K  T_nominal_value=1  Q_specify=off  Q_priority=None  Q=0 W  Q_nominal_specify=off  Q_nominal_unit=W  Q_nominal_value=1
      settings: SourceProductBaseCode=PW,SS,VE
  Brush Arm Conduction2 : fl_lib/Thermal/Thermal Elements/Conductive Heat Transfer  area=3*5 cm^2  thickness=4 cm  th_cond=1.7 W/(m*K)  T_specify=off  T_priority=None  T=0 K  T_nominal_specify=off  T_nominal_unit=K  T_nominal_value=1  Q_specify=off  Q_priority=None  Q=0 W  Q_nominal_specify=off  Q_nominal_unit=W  Q_nominal_value=1
      settings: SourceProductBaseCode=PW,SS,VE
  Case-Atmosphere Convection : fl_lib/Thermal/Thermal Elements/Convective Heat Transfer  area=4240 cm^2  heat_tr_coeff=26.8 W/(m^2 * K)  T_specify=off  T_priority=None  T=0 K  T_nominal_specify=off  T_nominal_unit=K  T_nominal_value=1  Q_specify=off  Q_priority=None  Q=0 W  Q_nominal_specify=off  Q_nominal_unit=W  Q_nominal_value=1
      settings: SourceProductBaseCode=PW,SS,VE
  Flange Thermal Mass : fl_lib/Thermal/Thermal Elements/Thermal Mass  mass=1.6 kg  sp_heat=447 J/kg/K  T_specify=off  T_priority=High  T=300 K  T_nominal_specify=off  T_nominal_unit=K  T_nominal_value=1  Q_specify=off  Q_priority=None  Q=0 W  Q_nominal_specify=off  Q_nominal_unit=W  Q_nominal_value=1
      settings: SourceProductBaseCode=PW,SS,VE
  Flange-Atmosphere Convection : fl_lib/Thermal/Thermal Elements/Convective Heat Transfer  area=324 cm^2  heat_tr_coeff=123.4 W/(m^2 * K)  T_specify=off  T_priority=None  T=0 K  T_nominal_specify=off  T_nominal_unit=K  T_nominal_value=1  Q_specify=off  Q_priority=None  Q=0 W  Q_nominal_specify=off  Q_nominal_unit=W  Q_nominal_value=1
      settings: SourceProductBaseCode=PW,SS,VE
  Motor Case Thermal Mass : fl_lib/Thermal/Thermal Elements/Thermal Mass  mass=3.8 kg  sp_heat=903 J/kg/K  T_specify=off  T_priority=High  T=300 K  T_nominal_specify=off  T_nominal_unit=K  T_nominal_value=1  Q_specify=off  Q_priority=None  Q=0 W  Q_nominal_specify=off  Q_nominal_unit=W  Q_nominal_value=1
      settings: SourceProductBaseCode=PW,SS,VE
  Permanent Magnet Thermal Mass : fl_lib/Thermal/Thermal Elements/Thermal Mass  mass=3.6 kg  sp_heat=447 J/kg/K  T_specify=off  T_priority=High  T=300 K  T_nominal_specify=off  T_nominal_unit=K  T_nominal_value=1  Q_specify=off  Q_priority=None  Q=0 W  Q_nominal_specify=off  Q_nominal_unit=W  Q_nominal_value=1
      settings: SourceProductBaseCode=PW,SS,VE
  Permanent Magnet -Case Conductance : fl_lib/Thermal/Thermal Elements/Conductive Heat Transfer  area=4350 cm^2  thickness=26 cm  th_cond=80.2 W/(m*K)  T_specify=off  T_priority=None  T=0 K  T_nominal_specify=off  T_nominal_unit=K  T_nominal_value=1  Q_specify=off  Q_priority=None  Q=0 W  Q_nominal_specify=off  Q_nominal_unit=W  Q_nominal_value=1
      settings: SourceProductBaseCode=PW,SS,VE
  Rotor-BearingF Conduction : fl_lib/Thermal/Thermal Elements/Conductive Heat Transfer  area=26.4 cm^2  thickness=2.5 cm  th_cond=80.2 W/(m*K)  T_specify=off  T_priority=None  T=0 K  T_nominal_specify=off  T_nominal_unit=K  T_nominal_value=1  Q_specify=off  Q_priority=None  Q=0 W  Q_nominal_specify=off  Q_nominal_unit=W  Q_nominal_value=1
      settings: SourceProductBaseCode=PW,SS,VE
  Rotor-BearingR Conduction : fl_lib/Thermal/Thermal Elements/Conductive Heat Transfer  area=26.4 cm^2  thickness=2.5 cm  th_cond=80.2 W/(m*K)  T_specify=off  T_priority=None  T=0 K  T_nominal_specify=off  T_nominal_unit=K  T_nominal_value=1  Q_specify=off  Q_priority=None  Q=0 W  Q_nominal_specify=off  Q_nominal_unit=W  Q_nominal_value=1
      settings: SourceProductBaseCode=PW,SS,VE
  Rotor-Case Convection : fl_lib/Thermal/Thermal Elements/Convective Heat Transfer  area=1240 cm^2  heat_tr_coeff=210 W/(m^2 * K)  T_specify=off  T_priority=None  T=0 K  T_nominal_specify=off  T_nominal_unit=K  T_nominal_value=1  Q_specify=off  Q_priority=None  Q=0 W  Q_nominal_specify=off  Q_nominal_unit=W  Q_nominal_value=1
      settings: SourceProductBaseCode=PW,SS,VE
  Wire-Case Conduction1 : fl_lib/Thermal/Thermal Elements/Conductive Heat Transfer  area=1 cm^2  thickness=0.2 cm  th_cond=4 W/(m*K)  T_specify=off  T_priority=None  T=0 K  T_nominal_specify=off  T_nominal_unit=K  T_nominal_value=1  Q_specify=off  Q_priority=None  Q=0 W  Q_nominal_specify=off  Q_nominal_unit=W  Q_nominal_value=1
      settings: SourceProductBaseCode=PW,SS,VE
  Wire-Case Conduction2 : fl_lib/Thermal/Thermal Elements/Conductive Heat Transfer  area=1 cm^2  thickness=0.2 cm  th_cond=4 W/(m*K)  T_specify=off  T_priority=None  T=0 K  T_nominal_specify=off  T_nominal_unit=K  T_nominal_value=1  Q_specify=off  Q_priority=None  Q=0 W  Q_nominal_specify=off  Q_nominal_unit=W  Q_nominal_value=1
      settings: SourceProductBaseCode=PW,SS,VE
  Wire1 : fl_lib/Thermal/Thermal Elements/Thermal Mass  mass=0.05 kg  sp_heat=385 J/kg/K  T_specify=off  T_priority=High  T=300 K  T_nominal_specify=off  T_nominal_unit=K  T_nominal_value=1  Q_specify=off  Q_priority=None  Q=0 W  Q_nominal_specify=off  Q_nominal_unit=W  Q_nominal_value=1
      settings: SourceProductBaseCode=PW,SS,VE
  Wire2 : fl_lib/Thermal/Thermal Elements/Thermal Mass  mass=0.05 kg  sp_heat=385 J/kg/K  T_specify=off  T_priority=High  T=300 K  T_nominal_specify=off  T_nominal_unit=K  T_nominal_value=1  Q_specify=off  Q_priority=None  Q=0 W  Q_nominal_specify=off  Q_nominal_unit=W  Q_nominal_value=1
      settings: SourceProductBaseCode=PW,SS,VE
  M : PMIOPort  Side=Right
  E : PMIOPort  Port=2  Side=Left
  connections:
  Wire2/LConn1 -- Wire-Case Conduction2/LConn1 -- Brush Arm Conduction2/RConn1
  Wire1/LConn1 -- Wire-Case Conduction1/LConn1 -- Brush Arm Conduction1/RConn1
  Brush Arm Conduction2/LConn1 -- Brush Arm Conduction1/LConn1 -- Brush Conduction/RConn1
  Permanent Magnet Thermal Mass/LConn1 -- Permanent Magnet -Case Conductance/LConn1
  Rotor-BearingR Conduction/LConn1 -- Rotor-BearingF Conduction/LConn1 -- M/RConn1 -- Brush Conduction/LConn1 -- Rotor-Case Convection/LConn1
  Bearing PlateF Thermal Mass/LConn1 -- Rotor-BearingF Conduction/RConn1 -- BearingF-Atmosphere Convection/LConn1 -- BearingF-Case Conduction/LConn1
  Flange Thermal Mass/LConn1 -- BearingR-Flange Conduction/RConn1 -- Flange-Atmosphere Convection/LConn1
  BearingR-Case Conduction/LConn1 -- BearingR-Flange Conduction/LConn1 -- Bearing PlateR Thermal Mass/LConn1 -- Rotor-BearingR Conduction/RConn1
  Rotor-Case Convection/RConn1 -- BearingR-Case Conduction/RConn1 -- BearingF-Case Conduction/RConn1 -- Wire-Case Conduction2/RConn1 -- Wire-Case Conduction1/RConn1 -- Permanent Magnet -Case Conductance/RConn1 -- Case-Atmosphere Convection/LConn1 -- Motor Case Thermal Mass/LConn1
  Case-Atmosphere Convection/RConn1 -- BearingF-Atmosphere Convection/RConn1 -- E/RConn1 -- Flange-Atmosphere Convection/RConn1

== system ssc_auto_ev_20b/Motor Drive ==
  iRef : Inport
  DC Motor1 : Subsystem  Tag=PublishSubsystem
      mask Display:
      | % Circle, in/out, and 'M'
      | image('ssc_dcmotor_maskicon.png');
      | 
      | % % Circle
      | % plot(sin(0:0.1:2.2*pi)*0.9,cos(0:0.1:2.2*pi)*0.9);
      | %
      | % % In/out
      | % plot([-1.3 -0.9],[0 0]);
      | % plot([1.3 0.9],[0 0]);
      | %
      | % % 'M'
      | % plot([0.5 0.5],[-0.5 0.5]);
      | % plot([-0.5 -0.5],[-0.5 0.5]);
      | % plot([0.5 0],[0.5 -0.5]);
      | % plot([-0.5 0],[0.5 -0.5]);
      | 
      | % Plot points to set plot range
      | color('white');plot(1.5,1.5);plot(-1.5,-1.5)
      | color('black');
      | 
      | port_label('RConn',1,'R');
      | port_label('RConn',2,'C');
      | port_label('LConn',1,'V+');
      | port_label('LConn',2,'V-');
  DC Motor2 : Subsystem  Tag=PublishSubsystem
      mask Display:
      | % Circle, in/out, and 'M'
      | image('ssc_dcmotor_maskicon.png');
      | 
      | % % Circle
      | % plot(sin(0:0.1:2.2*pi)*0.9,cos(0:0.1:2.2*pi)*0.9);
      | %
      | % % In/out
      | % plot([-1.3 -0.9],[0 0]);
      | % plot([1.3 0.9],[0 0]);
      | %
      | % % 'M'
      | % plot([0.5 0.5],[-0.5 0.5]);
      | % plot([-0.5 -0.5],[-0.5 0.5]);
      | % plot([0.5 0],[0.5 -0.5]);
      | % plot([-0.5 0],[0.5 -0.5]);
      | 
      | % Plot points to set plot range
      | color('white');plot(1.5,1.5);plot(-1.5,-1.5)
      | color('black');
      | 
      | port_label('RConn',1,'R');
      | port_label('RConn',2,'C');
      | port_label('LConn',1,'V+');
      | port_label('LConn',2,'V-');
  Ideal Rotational Motion Sensor : fl_lib/Mechanical/Mechanical Sensors/Ideal Rotational Motion Sensor  wrap_angle=simscape.enum.onoff.off  offset=0 rad
      settings: SourceProductBaseCode=PW,SS,VE
  MRRef : fl_lib/Mechanical/Rotational Elements/Mechanical Rotational Reference
      settings: SourceProductBaseCode=PW,SS,VE
  MRRef1 : fl_lib/Mechanical/Rotational Elements/Mechanical Rotational Reference
      settings: SourceProductBaseCode=PW,SS,VE
  MRRef2 : fl_lib/Mechanical/Rotational Elements/Mechanical Rotational Reference
      settings: SourceProductBaseCode=PW,SS,VE
  Motor Torque Controller 1 (System-Level Representation) : Subsystem
      settings: PortSchema="{\"entries\":[{\"content\":{\"sides\":[{\"content\":{\"connectorIds\":[\"LConn1\",\"LConn2\"]},\"type\":\"ConnectorPlacement.EquallySpacedRectSide\",\"uuid\":\"fa610323-4e51-4b68-84d8-5520af174050\"},{\"content\":{\"connectorIds\":[\"RConn1\",\"RConn2\"],\"side\":\"RIGHT\"},\"type\":\"ConnectorPlacement.EquallySpacedRectSide\",\"uuid\":\"4363b90b-a4e0-4b49-9dec-cc6d130d9345\"},{\"content\":{\"connectorIds\":[\"LConn3\"],\"side\":\"TOP\"},\"type\":\"ConnectorPlacement.EquallySpacedRectSide\",\"uuid\":\"1b5285b6-bf42-4633-bccd-78a8c0464c36\"}]},\"type\":\"ConnectorPlacement.EquallySpacedConnector\",\"uuid\":\"5522e717-4ae9-420d-ac3d-a671d244aac1\"}],\"packageUris\":[\"http://schema.mathworks.com/mf0/Connector/R2020b\"],\"version\":\"1.0\"}"
  Motor Torque Controller 1 (System-Level Representation)1 : Subsystem
      settings: PortSchema="{\"entries\":[{\"content\":{\"sides\":[{\"content\":{\"connectorIds\":[\"LConn1\",\"LConn2\"]},\"type\":\"ConnectorPlacement.EquallySpacedRectSide\",\"uuid\":\"fa610323-4e51-4b68-84d8-5520af174050\"},{\"content\":{\"connectorIds\":[\"RConn1\",\"RConn2\"],\"side\":\"RIGHT\"},\"type\":\"ConnectorPlacement.EquallySpacedRectSide\",\"uuid\":\"4363b90b-a4e0-4b49-9dec-cc6d130d9345\"},{\"content\":{\"connectorIds\":[\"LConn3\"],\"side\":\"TOP\"},\"type\":\"ConnectorPlacement.EquallySpacedRectSide\",\"uuid\":\"1b5285b6-bf42-4633-bccd-78a8c0464c36\"}]},\"type\":\"ConnectorPlacement.EquallySpacedConnector\",\"uuid\":\"5522e717-4ae9-420d-ac3d-a671d244aac1\"}],\"packageUris\":[\"http://schema.mathworks.com/mf0/Connector/R2020b\"],\"version\":\"1.0\"}"
  Sensing wMotor : Subsystem
      mask Display: disp('w');
  Simulink-PS G1 : nesl_utility/Simulink-PS Converter  PhysicalDomain=network_engine_domain  SubClassName=ps_input  LeftPortType=input  RightPortType=output  PseudoPeriodic=off  Frequencies=[]  NoiseDistribution=none  NoiseParameters=[]  Unit=A  AffineConversion=off  FilteringAndDerivatives=zero  SimscapeFilterOrder=1  InputFilterTimeConstant=1e-6  UdotUserProvided=1
      settings: SourceProductBaseCode=SS,PW,VE
  Winding-Iron Conductance/1 : fl_lib/Thermal/Thermal Elements/Conductive Heat Transfer  area=250 cm^2  thickness=0.2 cm  th_cond=360 W/(m*K)  T_specify=off  T_priority=None  T=0 K  T_nominal_specify=off  T_nominal_unit=K  T_nominal_value=1  Q_specify=off  Q_priority=None  Q=0 W  Q_nominal_specify=off  Q_nominal_unit=W  Q_nominal_value=1
      settings: SourceProductBaseCode=PW,SS,VE
  Winding-Iron Conductance/2 : fl_lib/Thermal/Thermal Elements/Conductive Heat Transfer  area=250 cm^2  thickness=0.2 cm  th_cond=360 W/(m*K)  T_specify=off  T_priority=None  T=0 K  T_nominal_specify=off  T_nominal_unit=K  T_nominal_value=1  Q_specify=off  Q_priority=None  Q=0 W  Q_nominal_specify=off  Q_nominal_unit=W  Q_nominal_value=1
      settings: SourceProductBaseCode=PW,SS,VE
  + : PMIOPort  Side=Left
  - : PMIOPort  Port=2  Side=Left
  R : PMIOPort  Port=3  Side=Right
  M1 : PMIOPort  Port=4  Side=Left
  M2 : PMIOPort  Port=5  Side=Left
  w : Outport  VectorParamsAs1DForOutWhenUnconnected=off
  wires:
  Sensing wMotor/1(SL) -> w/1
  iRef/1 -> Simulink-PS G1/1
  connections:
  Ideal Rotational Motion Sensor/RConn2 -- Sensing wMotor/LConn1
  DC Motor1/RConn1 -- DC Motor2/RConn1 -- Ideal Rotational Motion Sensor/LConn1 -- R/RConn1
  DC Motor1/RConn2 -- MRRef/LConn1
  MRRef1/LConn1 -- Ideal Rotational Motion Sensor/RConn1
  Motor Torque Controller 1 (System-Level Representation)/LConn1 -- DC Motor1/LConn1
  +/RConn1 -- Motor Torque Controller 1 (System-Level Representation)1/RConn1 -- Motor Torque Controller 1 (System-Level Representation)/RConn1
  -/RConn1 -- Motor Torque Controller 1 (System-Level Representation)1/RConn2 -- Motor Torque Controller 1 (System-Level Representation)/RConn2
  DC Motor1/LConn2 -- Motor Torque Controller 1 (System-Level Representation)/LConn2
  Simulink-PS G1/RConn1 -- Motor Torque Controller 1 (System-Level Representation)/LConn3 -- Motor Torque Controller 1 (System-Level Representation)1/LConn3
  DC Motor2/RConn2 -- MRRef2/LConn1
  DC Motor2/LConn1 -- Motor Torque Controller 1 (System-Level Representation)1/LConn1
  DC Motor2/LConn2 -- Motor Torque Controller 1 (System-Level Representation)1/LConn2
  Winding-Iron Conductance/1/RConn1 -- DC Motor1/LConn3
  Winding-Iron Conductance/2/RConn1 -- DC Motor2/LConn3
  M1/RConn1 -- Winding-Iron Conductance/1/LConn1
  M2/RConn1 -- Winding-Iron Conductance/2/LConn1
